simulink model "Regulator23a"  (R2023a)
settings: Solver=FixedStepDiscrete  StartTime=0.0  StopTime=10.0  FixedStep=0.005  RelTol=1e-3
settings Model: Creator=andriyanov_ilya  LastModifiedBy=Ilya_Andriyanov

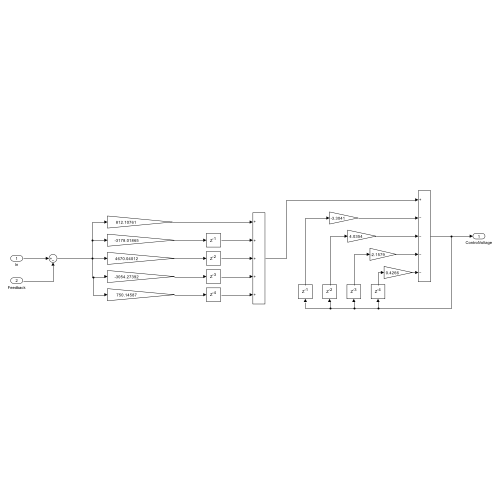
[thumbnail: Simulink's stored preview of the top-level diagram]
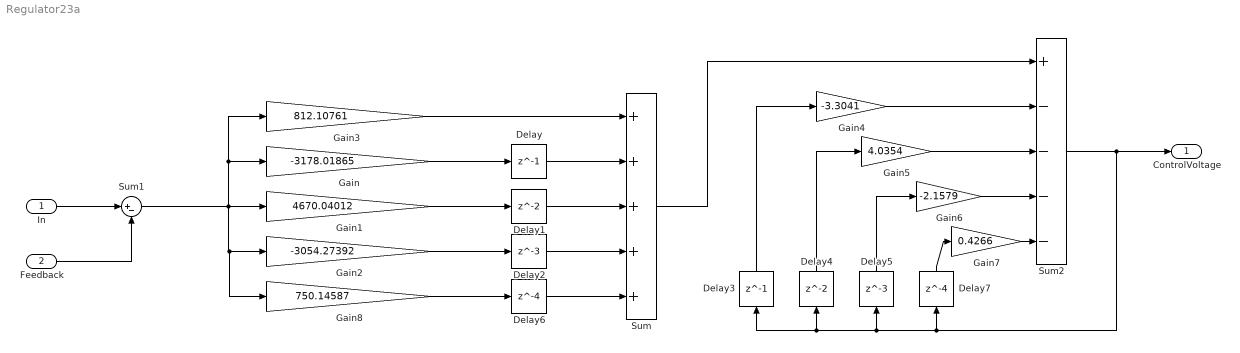
== system Regulator23a ==
  In : Inport
  Feedback : Inport  Port=2
  Delay : Delay  DelayLength=1
  Delay1 : Delay
  Delay2 : Delay  DelayLength=3
  Delay3 : Delay  DelayLength=1
  Delay4 : Delay
  Delay5 : Delay  DelayLength=3
  Delay6 : Delay  DelayLength=4
  Delay7 : Delay  DelayLength=4
  Gain : Gain  Gain=-3178.01865
  Gain1 : Gain  Gain=4670.04012
  Gain2 : Gain  Gain=-3054.27392
  Gain3 : Gain  Gain=812.10761
  Gain4 : Gain  Gain=-3.3041
  Gain5 : Gain  Gain=4.0354
  Gain6 : Gain  Gain=-2.1579
  Gain7 : Gain  Gain=0.4266
  Gain8 : Gain  Gain=750.14587
  Sum : Sum  Inputs=+++++
  Sum1 : Sum  Inputs=|+-
  Sum2 : Sum  Inputs=+----
  ControlVoltage : Outport
  wires:
  In/1 -> Sum1/1
  Feedback/1 -> Sum1/2
  Gain7/1 -> Sum2/5
  Delay7/1 -> Gain7/1
  Delay/1 -> Sum/2
  Delay1/1 -> Sum/3
  Delay5/1 -> Gain6/1
  Gain8/1 -> Delay6/1
  Gain4/1 -> Sum2/2
  Gain3/1 -> Sum/1
  Gain/1 -> Delay/1
  Delay4/1 -> Gain5/1
  Gain2/1 -> Delay2/1
  Gain1/1 -> Delay1/1
  Delay2/1 -> Sum/4
  Gain6/1 -> Sum2/4
  Sum/1 -> Sum2/1
  Delay6/1 -> Sum/5
  Delay3/1 -> Gain4/1
  Gain5/1 -> Sum2/3
  Sum1/1 -> Gain3/1, Gain/1, Gain8/1, Gain2/1, Gain1/1
  Sum2/1 -> ControlVoltage/1, Delay4/1, Delay3/1, Delay5/1, Delay7/1
